simulink model "uav_control_fb_lin_lqr"  (R2023a)
settings: Solver=FixedStepAuto  StartTime=0.0  StopTime=50  FixedStep=1e-3
undefined symbols (not defined in the file): b, d, g, J1, J2, J3, K_lqr, L, m, Matrix_Force2angular_velocity
libraries: simulink x22, hamilton x1, lagrange x1, control_form_NL x1, control_form_NL_forces x1
(part 1 of 2)
settings Model: Creator=Alex  LastModifiedBy=Alex

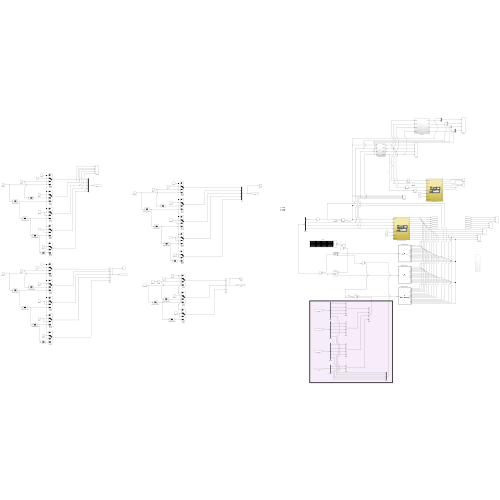
[thumbnail: Simulink's stored preview of the top-level diagram]
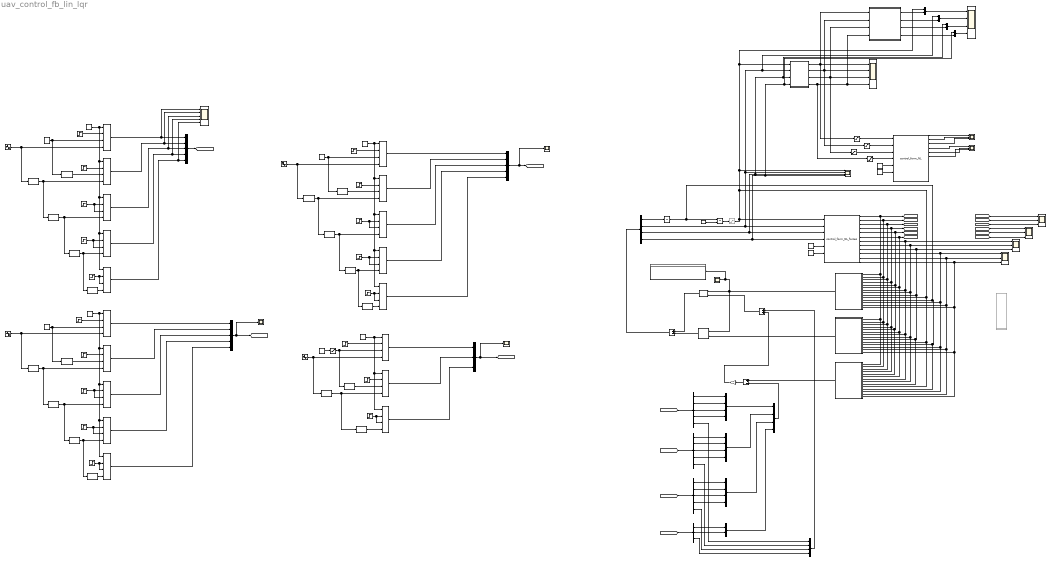
== system uav_control_fb_lin_lqr ==
  note: 1 - step
      | 2 - ramp
      | 3 - else
  Add : Sum  Inputs=+-
  Add1 : Sum  Inputs=+-
  Add2 : Sum
  CNL_AngPos : Scope  NumInputPorts=3
  CNL_AngVel : Scope  NumInputPorts=3
  CNL_LinPos : Scope  NumInputPorts=3
  CNL_LinVel : Scope  NumInputPorts=3
  Constant1 : Constant  Value=[1 0 0 0 1 1 0]
  Constant2 : Constant  Value=[1 1 -1 0 0 0 0 0 0 0 0 0 ]
  Constant3 : Constant  Value=1e-3
  Constant4 : Constant  Value=[1 0 0 0 1 1 0]
  Constant5 : Constant  Value=[1 1 -1 0 0 0 0 0 0 0 0 0 ]
  Demux : Demux
  Demux1 : Demux  Outputs=5
  Demux2 : Demux  Outputs=5
  Demux3 : Demux  Outputs=5
  Demux4 : Demux  Outputs=3
  Discrete Derivative{,1..17} (18 alike) : simulink/Discrete/Discrete Derivative  gainval=1.0  ICPrevScaledInput=0.0  OutMin=[]  OutMax=[]  OutDataType=fixdt(1, 16)  OutScaling=2^-10  DoSatur=off
  Display : Display
  Force2AngularVelocity : Subsystem
  Gain1 : Gain  Gain=-K_lqr  Multiplication=Matrix(K*u)
  Input_psi : Constant
  Input_x : Constant
  Input_y : Constant
  Input_z : Constant
  Integrator : Integrator
  Integrator1 : Integrator  InitialConditionSource=external
  MATLAB Function : MATLAB Function  TreatAsAtomicUnit=on
  MATLAB Function1 : MATLAB Function  TreatAsAtomicUnit=on
  MATLAB Function2 : MATLAB Function  TreatAsAtomicUnit=on
  Matrix Multiply : Product  Multiplication=Matrix(*)
  Multiport Switch{,1..17} (18 alike) : MultiPortSwitch  SaturateOnIntegerOverflow=off  InputSameDT=off
  Mux : Mux  Inputs=5
  Mux1 : Mux  Inputs=5
  Mux{8,10..13} (5 alike) : Mux  Inputs=2
  Mux{2,4,6..7,9} (5 alike) : Mux
  Mux3 : Mux  Inputs=3
  Mux5 : Mux  Inputs=5
  Product : Product  Multiplication=Matrix(*)
  Ramp_psi : simulink/Sources/Ramp  slope=0.2  start=0  InitialOutput=0
  Ramp_x : simulink/Sources/Ramp  slope=1  start=0  InitialOutput=1
  Ramp_y : simulink/Sources/Ramp  slope=1  start=0  InitialOutput=0
  Ramp_z : simulink/Sources/Ramp  slope=-5  start=0  InitialOutput=0
  STEP0_{1..14} (14 alike) : Step  Time=0  After=0  SampleTime=0
  Saturation : Saturate  UpperLimit=pi  LowerLimit=-pi
  Saturation1 : Saturate  Commented=through  UpperLimit=inf  LowerLimit=0
  Saturation{2..5} (4 alike) : Saturate  UpperLimit=1000  LowerLimit=0
  Scope{,2..4} (4 alike) : Scope
  Scope1 : Scope  NumInputPorts=5
  Scope5 : Scope  NumInputPorts=4
  Scope6 : Scope  NumInputPorts=3
  Scope7 : Scope  NumInputPorts=3
  Scope8 : Scope  NumInputPorts=4
  Scope9 : Scope  NumInputPorts=4
  Sine Wave_psi : Sin  SampleTime=0
  Sine Wave_x : Sin  Frequency=0.5  SampleTime=0
  Sine Wave_y : Sin  Amplitude=3  Bias=5  SampleTime=0
  Sine Wave_z : Sin  Amplitude=3  Bias=-5  SampleTime=0
  Step_psi : Step  Time=0  SampleTime=0
  Step_x : Step  Time=0  After=5  SampleTime=0
  Step_y : Step  Time=0  After=5  SampleTime=0
  Step_z : Step  Time=0  After=-7  SampleTime=0
  Subsystem : Subsystem  Commented=on
  Subsystem1 : Subsystem
  control_form_NL : control_form_NL/control_form_NL  SystemSampleTime=-1  VariantActivationTime=update diagram  Latency=0  AutoFrameSizeCalculation=off
  control_form_NL_forces : control_form_NL_forces/control_form_NL_forces  SystemSampleTime=-1  VariantActivationTime=update diagram  Latency=0  AutoFrameSizeCalculation=off
      settings: LibrarySourceBlock=control_form_NL_forces/control_form_NL
  wires:
  control_form_NL_forces/3 -> MATLAB Function2/3(z), MATLAB Function1/3(z), MATLAB Function/3(z), [CNL_z]
  control_form_NL_forces/2 -> MATLAB Function2/2(y), MATLAB Function1/2(y), MATLAB Function/2(y), [CNL_y]
  control_form_NL_forces/1 -> MATLAB Function2/1(x), MATLAB Function1/1(x), MATLAB Function/1(x), [CNL_x]
  control_form_NL_forces/4 -> MATLAB Function2/4(phi), MATLAB Function1/4(phi), MATLAB Function/4(phi), [CNL_phi]
  control_form_NL_forces/5 -> MATLAB Function2/5(theta), MATLAB Function1/5(theta), MATLAB Function/5(theta), [CNL_theta]
  control_form_NL_forces/6 -> MATLAB Function2/6(psi), MATLAB Function1/6(psi), MATLAB Function/6(psi), [CNL_psi]
  [CNL_x] -> CNL_LinPos/1
  [CNL_y] -> CNL_LinPos/2
  [CNL_z] -> CNL_LinPos/3
  [CNL_phi] -> CNL_AngPos/1
  [CNL_theta] -> CNL_AngPos/2
  [CNL_psi] -> CNL_AngPos/3
  control_form_NL_forces/7 -> MATLAB Function2/7(xdot), MATLAB Function1/7(xdot), MATLAB Function/7(xdot), CNL_LinVel/1
  control_form_NL_forces/8 -> MATLAB Function2/8(ydot), MATLAB Function1/8(ydot), MATLAB Function/8(ydot), CNL_LinVel/2
  control_form_NL_forces/9 -> MATLAB Function/9(zdot), MATLAB Function2/9(zdot), MATLAB Function1/9(zdot), CNL_LinVel/3
  control_form_NL_forces/10 -> CNL_AngVel/1, MATLAB Function2/12(p), MATLAB Function1/12(p), MATLAB Function/12(p)
  control_form_NL_forces/11 -> CNL_AngVel/2, MATLAB Function2/13(q), MATLAB Function1/13(q), MATLAB Function/13(q)
  control_form_NL_forces/12 -> CNL_AngVel/3, MATLAB Function2/14(r), MATLAB Function1/14(r), MATLAB Function/14(r)
  Integrator/1 -> MATLAB Function/11(xi), MATLAB Function2/11(xi), MATLAB Function1/11(xi), Integrator1/1  "xi"
  Product/1 -> Add/2  "alpha"
  MATLAB Function1/1(b) -> Product/2
  MATLAB Function/1(delta_inv) -> Display/1, Scope/1, Matrix Multiply/1, Product/1  "beta"
  Matrix Multiply/1 -> Add/1
  Add1/1 -> Gain1/1  "z"
  Gain1/1 -> Add2/2  "v"
  Add/1 -> Demux/1
  Demux/1 -> Integrator/1  "u1_tilde"
  Integrator1/1 -> Saturation1/1  "zeta"
  Step_x/1 -> Multiport Switch/2
  Mux/1 -> [xref]
  Constant1/1 -> control_form_NL_forces/6
  Constant2/1 -> control_form_NL_forces/5
  Constant3/1 -> Integrator1/2
  Mux1/1 -> [yref], Scope2/1
  Step_psi/1 -> Multiport Switch15/2
  Mux3/1 -> [psiref], Scope4/1
  MATLAB Function2/1(transf) -> Add1/1  "z"
  Mux4/1 -> Add1/2
  Ramp_x/1 -> Discrete Derivative/1, Multiport Switch/3
  Sine Wave_x/1 -> Multiport Switch/4, Discrete Derivative1/1
  Input_x/1 -> Multiport Switch4/1, Multiport Switch3/1, Multiport Switch2/1, Multiport Switch1/1, Multiport Switch/1
  STEP0_1/1 -> Multiport Switch1/2
  Discrete Derivative/1 -> Multiport Switch1/3
  Discrete Derivative1/1 -> Multiport Switch1/4, Discrete Derivative2/1
  STEP0_2/1 -> Multiport Switch2/3, Multiport Switch2/2
  Discrete Derivative2/1 -> Multiport Switch2/4, Discrete Derivative3/1
  STEP0_3/1 -> Multiport Switch3/3, Multiport Switch3/2
  Discrete Derivative3/1 -> Multiport Switch3/4, Discrete Derivative4/1
  Discrete Derivative4/1 -> Multiport Switch4/4
  STEP0_4/1 -> Multiport Switch4/3, Multiport Switch4/2
  Multiport Switch/1 -> Mux/1, Scope1/1
  Multiport Switch1/1 -> Mux/2, Scope1/2
  Multiport Switch2/1 -> Mux/3, Scope1/3
  Multiport Switch3/1 -> Mux/4, Scope1/4
  Multiport Switch4/1 -> Scope1/5, Mux/5
  Multiport Switch9/1 -> Mux1/5
  Multiport Switch8/1 -> Mux1/4
  Multiport Switch7/1 -> Mux1/3
  Multiport Switch6/1 -> Mux1/2
  Multiport Switch5/1 -> Mux1/1
  STEP0_8/1 -> Multiport Switch9/2, Multiport Switch9/3
  Discrete Derivative9/1 -> Multiport Switch9/4
  Discrete Derivative8/1 -> Discrete Derivative9/1, Multiport Switch8/4
  STEP0_7/1 -> Multiport Switch8/2, Multiport Switch8/3
  Discrete Derivative7/1 -> Discrete Derivative8/1, Multiport Switch7/4
  STEP0_6/1 -> Multiport Switch7/2, Multiport Switch7/3
  Discrete Derivative6/1 -> Discrete Derivative7/1, Multiport Switch6/4
  Discrete Derivative5/1 -> Multiport Switch6/3
  STEP0_5/1 -> Multiport Switch6/2
  Input_y/1 -> Multiport Switch5/1, Multiport Switch6/1, Multiport Switch7/1, Multiport Switch8/1, Multiport Switch9/1
  Sine Wave_y/1 -> Discrete Derivative6/1, Multiport Switch5/4
  Ramp_y/1 -> Multiport Switch5/3, Discrete Derivative5/1
  Step_y/1 -> Multiport Switch5/2
  Step_z/1 -> Multiport Switch10/2
  Ramp_z/1 -> Discrete Derivative10/1, Multiport Switch10/3
  Sine Wave_z/1 -> Multiport Switch10/4, Discrete Derivative11/1
  Input_z/1 -> Multiport Switch14/1, Multiport Switch13/1, Multiport Switch12/1, Multiport Switch11/1, Multiport Switch10/1
  STEP0_9/1 -> Multiport Switch11/2
  Discrete Derivative10/1 -> Multiport Switch11/3
  Discrete Derivative11/1 -> Multiport Switch11/4, Discrete Derivative12/1
  STEP0_10/1 -> Multiport Switch12/3, Multiport Switch12/2
  Discrete Derivative12/1 -> Multiport Switch12/4, Discrete Derivative13/1
  STEP0_11/1 -> Multiport Switch13/3, Multiport Switch13/2
  Discrete Derivative13/1 -> Multiport Switch13/4, Discrete Derivative14/1
  Discrete Derivative14/1 -> Multiport Switch14/4
  STEP0_12/1 -> Multiport Switch14/3, Multiport Switch14/2
  Multiport Switch10/1 -> Mux5/1
  Multiport Switch11/1 -> Mux5/2
  Multiport Switch12/1 -> Mux5/3
  Multiport Switch13/1 -> Mux5/4
  Multiport Switch14/1 -> Mux5/5
  Mux5/1 -> Scope3/1, [zref]
  Input_psi/1 -> Multiport Switch17/1, Multiport Switch16/1, Multiport Switch15/1
  Ramp_psi/1 -> Saturation/1
  Saturation/1 -> Discrete Derivative15/1, Multiport Switch15/3
  Sine Wave_psi/1 -> Discrete Derivative16/1, Multiport Switch15/4
  STEP0_13/1 -> Multiport Switch16/2
  Discrete Derivative15/1 -> Multiport Switch16/3
  Discrete Derivative16/1 -> Discrete Derivative17/1, Multiport Switch16/4
  STEP0_14/1 -> Multiport Switch17/3, Multiport Switch17/2
  Discrete Derivative17/1 -> Multiport Switch17/4
  [xref] -> Demux1/1
  Demux1/1 -> Mux2/1
  Demux1/2 -> Mux2/2
  Demux1/3 -> Mux2/3
  Demux1/4 -> Mux2/4
  Mux2/1 -> Mux4/1
  Mux6/1 -> Mux4/2
  Demux2/4 -> Mux6/4
  Demux2/3 -> Mux6/3
  Demux2/2 -> Mux6/2
  Demux2/1 -> Mux6/1
  [yref] -> Demux2/1
  [zref] -> Demux3/1
  Demux3/1 -> Mux7/1
  Demux3/2 -> Mux7/2
  Demux3/3 -> Mux7/3
  Demux3/4 -> Mux7/4
  Mux7/1 -> Mux4/3
  [psiref] -> Demux4/1
  Demux4/1 -> Mux8/1
  Demux4/2 -> Mux8/2
  Mux8/1 -> Mux4/4
  Demux4/3 -> Mux9/4
  Demux3/5 -> Mux9/3
  Demux2/5 -> Mux9/2
  Demux1/5 -> Mux9/1
  Mux9/1 -> Add2/1
  Add2/1 -> Matrix Multiply/2
  Constant5/1 -> control_form_NL/5
  Constant4/1 -> control_form_NL/6
  control_form_NL/1 -> Scope6/1
  control_form_NL/2 -> Scope6/2
  control_form_NL/3 -> Scope6/3
  control_form_NL/4 -> Scope7/1
  control_form_NL/5 -> Scope7/2
  control_form_NL/6 -> Scope7/3
  Force2AngularVelocity/1(omega_f) -> Subsystem1/1(omega_f), Scope8/1, Saturation2/1  "front"
  Force2AngularVelocity/2(omega_b) -> Subsystem1/2(omega_b), Scope8/2, Saturation3/1  "back"
  Force2AngularVelocity/3(omega_l) -> Subsystem1/3(omega_l), Scope8/3, Saturation4/1  "left"
  Force2AngularVelocity/4(omega_r) -> Saturation5/1, Subsystem1/4(omega_r), Scope8/4  "right"
  Demux/4 -> control_form_NL_forces/4, Mux13/1, Force2AngularVelocity/4(u4), Scope5/4
  Demux/3 -> control_form_NL_forces/3, Mux12/1, Force2AngularVelocity/3(u3), Scope5/3
  Demux/2 -> control_form_NL_forces/2, Mux11/1, Force2AngularVelocity/2(u2), Scope5/2
  Multiport Switch15/1 -> Mux3/1
  Multiport Switch16/1 -> Mux3/2
  Multiport Switch17/1 -> Mux3/3
  Saturation1/1 -> control_form_NL_forces/1, MATLAB Function2/10(zeta), MATLAB Function1/10(zeta), MATLAB Function/10(zeta), Mux10/1, Force2AngularVelocity/1(u1), Scope5/1
  Subsystem1/1(Thrust) -> Mux10/2
  Subsystem1/2(M1) -> Mux11/2
  Subsystem1/3(M2) -> Mux12/2
  Subsystem1/4(M3) -> Mux13/2
  Mux13/1 -> Scope9/4
  Mux12/1 -> Scope9/3
  Mux11/1 -> Scope9/2
  Mux10/1 -> Scope9/1
  Saturation2/1 -> control_form_NL/1
  Saturation3/1 -> control_form_NL/2
  Saturation4/1 -> control_form_NL/3
  Saturation5/1 -> control_form_NL/4

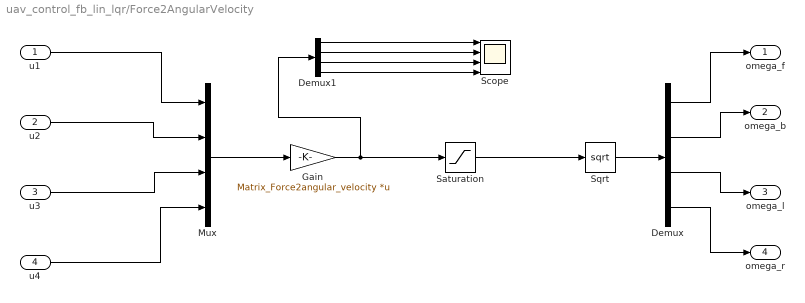
== system uav_control_fb_lin_lqr/Force2AngularVelocity ==
  u1 : Inport
  u2 : Inport  Port=2
  u3 : Inport  Port=3
  u4 : Inport  Port=4
  Demux : Demux
  Demux1 : Demux
  Gain : Gain  Gain=Matrix_Force2angular_velocity  Multiplication=Matrix(K*u)
  Mux : Mux
  Saturation : Saturate  UpperLimit=inf  LowerLimit=0
  Scope : Scope  NumInputPorts=4
  Sqrt : Sqrt
  omega_f : Outport
  omega_b : Outport  Port=2
  omega_l : Outport  Port=3
  omega_r : Outport  Port=4
  wires:
  u3/1 -> Mux/3
  u2/1 -> Mux/2
  u4/1 -> Mux/4
  u1/1 -> Mux/1
  Mux/1 -> Gain/1
  Sqrt/1 -> Demux/1
  Demux/3 -> omega_l/1
  Demux/2 -> omega_b/1
  Demux/4 -> omega_r/1
  Demux/1 -> omega_f/1
  Demux1/1 -> Scope/1
  Demux1/2 -> Scope/2
  Demux1/3 -> Scope/3
  Demux1/4 -> Scope/4
  Gain/1 -> Saturation/1, Demux1/1
  Saturation/1 -> Sqrt/1

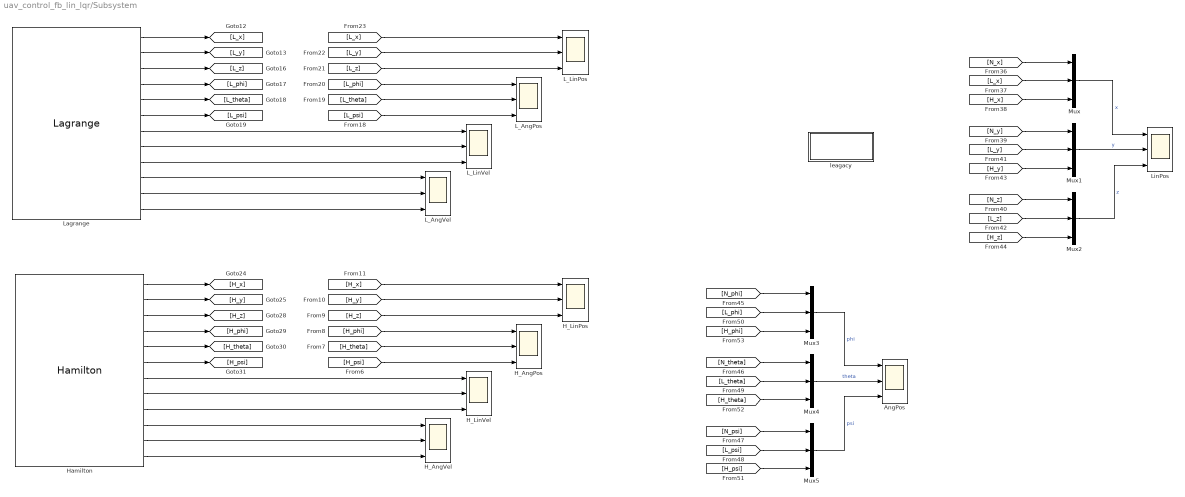
== system uav_control_fb_lin_lqr/Subsystem ==
  AngPos : Scope  NumInputPorts=3
  H_AngPos : Scope  NumInputPorts=3
  H_AngVel : Scope  NumInputPorts=3
  H_LinPos : Scope  NumInputPorts=3
  H_LinVel : Scope  NumInputPorts=3
  Hamilton : hamilton/Hamilton  SystemSampleTime=-1  VariantActivationTime=update diagram  Latency=0  AutoFrameSizeCalculation=off
  L_AngPos : Scope  NumInputPorts=3
  L_AngVel : Scope  NumInputPorts=3
  L_LinPos : Scope  NumInputPorts=3
  L_LinVel : Scope  NumInputPorts=3
  Lagrange : lagrange/Lagrange  SystemSampleTime=-1  VariantActivationTime=update diagram  Latency=0  AutoFrameSizeCalculation=off
  LinPos : Scope  NumInputPorts=3
  Mux{,1..5} (6 alike) : Mux  Inputs=3
  leagacy : Subsystem
  wires:
  Hamilton/2 -> [H_y]
  Mux4/1 -> AngPos/2  "theta"
  [H_theta] -> Mux4/3
  Hamilton/1 -> [H_x]
  Lagrange/11 -> L_AngVel/2
  Mux3/1 -> AngPos/1  "phi"
  [H_theta] -> H_AngPos/2
  Lagrange/4 -> [L_phi]
  Hamilton/6 -> [H_psi]
  Hamilton/10 -> H_AngVel/1
  [H_z] -> H_LinPos/3
  [H_y] -> H_LinPos/2
  Lagrange/10 -> L_AngVel/1
  Lagrange/2 -> [L_y]
  Lagrange/5 -> [L_theta]
  [L_theta] -> Mux4/2
  Hamilton/3 -> [H_z]
  [L_psi] -> Mux5/2
  Lagrange/9 -> L_LinVel/3
  Lagrange/6 -> [L_psi]
  Hamilton/5 -> [H_theta]
  Hamilton/11 -> H_AngVel/2
  Hamilton/9 -> H_LinVel/3
  [L_phi] -> L_AngPos/1
  Lagrange/8 -> L_LinVel/2
  [L_psi] -> L_AngPos/3
  Lagrange/7 -> L_LinVel/1
  [H_psi] -> H_AngPos/3
  [H_psi] -> Mux5/3
  [H_x] -> H_LinPos/1
  [N_psi] -> Mux5/1
  Hamilton/8 -> H_LinVel/2
  [L_x] -> L_LinPos/1
  Hamilton/4 -> [H_phi]
  [L_z] -> L_LinPos/3
  [L_y] -> L_LinPos/2
  Hamilton/12 -> H_AngVel/3
  Mux5/1 -> AngPos/3  "psi"
  Hamilton/7 -> H_LinVel/1
  [H_phi] -> Mux3/3
  Lagrange/12 -> L_AngVel/3
  Lagrange/3 -> [L_z]
  [L_phi] -> Mux3/2
  [N_theta] -> Mux4/1
  [N_phi] -> Mux3/1
  Lagrange/1 -> [L_x]
  [L_theta] -> L_AngPos/2
  [H_phi] -> H_AngPos/1
  [N_x] -> Mux/1
  Mux2/1 -> LinPos/3  "z"
  [H_x] -> Mux/3
  Mux/1 -> LinPos/1  "x"
  [N_z] -> Mux2/1
  [L_x] -> Mux/2
  [L_y] -> Mux1/2
  [L_z] -> Mux2/2
  [N_y] -> Mux1/1
  [H_z] -> Mux2/3
  Mux1/1 -> LinPos/2  "y"
  [H_y] -> Mux1/3

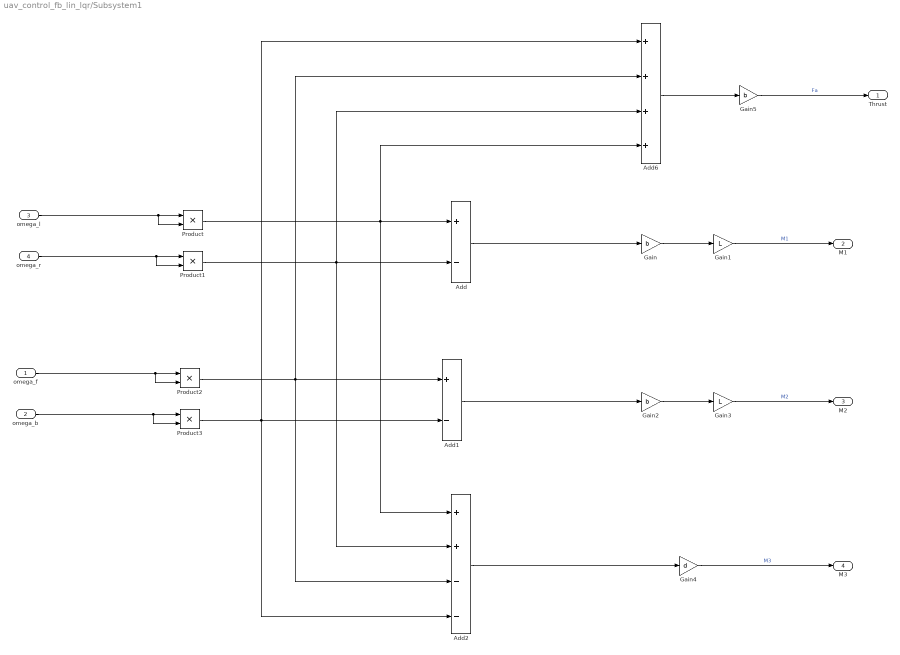
== system uav_control_fb_lin_lqr/Subsystem1 ==
  omega_f : Inport
  omega_b : Inport  Port=2
  omega_l : Inport  Port=3
  omega_r : Inport  Port=4
  Add : Sum  Inputs=+-
  Add1 : Sum  Inputs=+-
  Add2 : Sum  Inputs=++--
  Add6 : Sum  Inputs=++++
  Gain : Gain  Gain=b
  Gain1 : Gain  Gain=L
  Gain2 : Gain  Gain=b
  Gain3 : Gain  Gain=L
  Gain4 : Gain  Gain=d
  Gain5 : Gain  Gain=b
  Product{,1..3} (4 alike) : Product
  Thrust : Outport
  M1 : Outport  Port=2
  M2 : Outport  Port=3
  M3 : Outport  Port=4
  wires:
  Add/1 -> Gain/1
  Gain2/1 -> Gain3/1
  omega_b/1 -> Product3/1, Product3/2
  Product3/1 -> Add6/1, Add2/4, Add1/2
  Product/1 -> Add6/4, Add2/1, Add/1
  omega_f/1 -> Product2/1, Product2/2
  omega_r/1 -> Product1/1, Product1/2
  Add1/1 -> Gain2/1
  Gain4/1 -> M3/1  "M3"
  Add2/1 -> Gain4/1
  Product1/1 -> Add6/3, Add2/2, Add/2
  omega_l/1 -> Product/1, Product/2
  Gain3/1 -> M2/1  "M2"
  Product2/1 -> Add6/2, Add2/3, Add1/1
  Gain/1 -> Gain1/1
  Gain1/1 -> M1/1  "M1"
  Add6/1 -> Gain5/1
  Gain5/1 -> Thrust/1  "Fa"

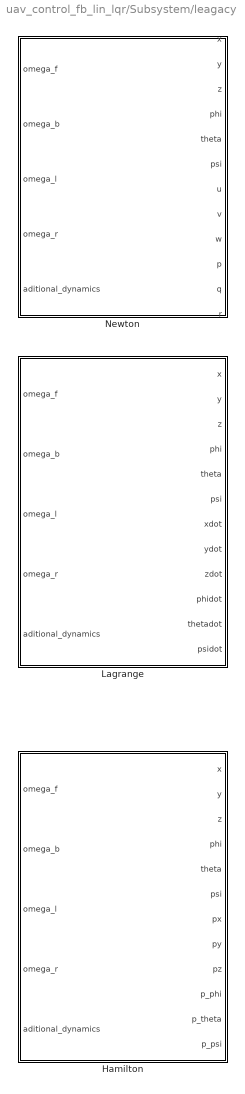
== system uav_control_fb_lin_lqr/Subsystem/leagacy ==
  Hamilton : Subsystem
  Lagrange : Subsystem
  Newton : Subsystem

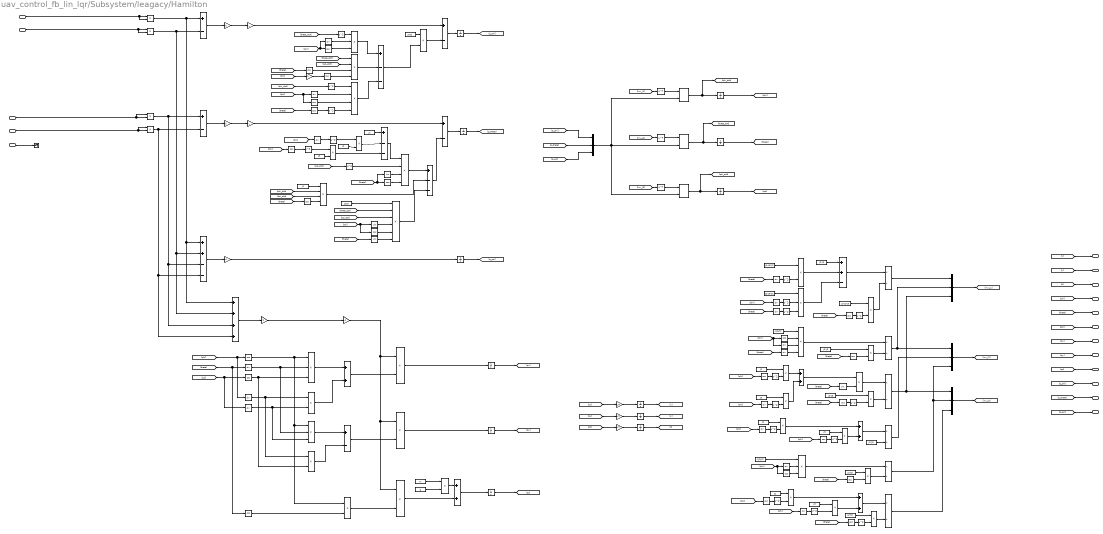
== system uav_control_fb_lin_lqr/Subsystem/leagacy/Hamilton ==
  note: F_thrust
  note: Rotational generalized coordinates (positions)
  note: Translational generalized coordinates (positions)
  note: Translational momentum equations
  note: Rotational momentum equations
  note: Matrix J^(-1) computation
  omega_f : Inport
  omega_b : Inport  Port=2
  omega_l : Inport  Port=3
  omega_r : Inport  Port=4
  aditional_dynamics : Inport  Port=5
  Add{,1,3..4,11} (5 alike) : Sum  Inputs=+-
  Add{10,14,26..28} (5 alike) : Sum
  Add2 : Sum  Inputs=++--
  Add25 : Sum  Inputs=++-
  Add5 : Sum  Inputs=+--
  Add6 : Sum  Inputs=++++
  Add7 : Sum  Inputs=+--
  Add8 : Sum  Inputs=+--
  Constant1 : Constant  Value=J3-J2
  Constant2 : Constant  Value=J1
  Constant{22,26,28,31,34,36} (6 alike) : Constant  Value=J2*J3
  Constant23 : Constant  Value=(J1-J3)*J2
  Constant24 : Constant  Value=(J2-J3)*J1
  Constant25 : Constant  Value=J1*J2*J3
  Constant27 : Constant  Value=-(J2-J3)
  Constant{3,29,32,37} (4 alike) : Constant  Value=J2
  Constant{8,30,33,38} (4 alike) : Constant  Value=J3
  Constant35 : Constant  Value=-(J2-J3)
  Constant4 : Constant  Value=J1
  Constant5 : Constant  Value=J2-J3
  Constant6 : Constant  Value=m
  Constant7 : Constant  Value=g
  Cos{,1,3,5,7,53..55,58,60,63..64,66..67,69} (15 alike) : Trigonometry  Operator=cos
  Cos{4,6,8,50..52,56..57,59,61..62,65,68} (13 alike) : Trigonometry
  Divide{6..11} (6 alike) : Product  Inputs=*/
  Gain : Gain  Gain=b
  Gain1 : Gain  Gain=L
  Gain10 : Gain  Gain=-1
  Gain2 : Gain  Gain=b
  Gain3 : Gain  Gain=L
  Gain4 : Gain  Gain=d
  Gain5 : Gain  Gain=b
  Gain6 : Gain  Gain=1/m
  Gain7 : Gain  Gain=1/m
  Gain8 : Gain  Gain=1/m
  Gain9 : Gain  Gain=2
  Integrator{,1..11} (12 alike) : Integrator
  Matrix Multiply1 : Product  Multiplication=Matrix(*)
  Matrix Multiply2 : Product  Multiplication=Matrix(*)
  Matrix Multiply5 : Product  Multiplication=Matrix(*)
  Mux{,7..9} (4 alike) : Mux  Inputs=3
  Product{,1..4,11..12,14,16..21,44,46..47,49..55,57..59} (27 alike) : Product
  Product10 : Product  Inputs=6
  Product{5,13,15,45,56} (5 alike) : Product  Inputs=3
  Product{6..9,48} (5 alike) : Product  Inputs=4
  Sin{,4,7..10} (6 alike) : Trigonometry
  Sin{1..3,5..6,11..12} (7 alike) : Trigonometry  Operator=cos
  Square{1..6,13..24} (18 alike) : Math  Operator=square
  Terminator : Terminator
  Transpose1 : Math  Operator=transpose
  Transpose2 : Math  Operator=transpose
  Transpose5 : Math  Operator=transpose
  x : Outport
  y : Outport  Port=2
  z : Outport  Port=3
  phi : Outport  Port=4
  theta : Outport  Port=5
  psi : Outport  Port=6
  px : Outport  Port=7
  py : Outport  Port=8
  pz : Outport  Port=9
  p_phi : Outport  Port=10
  p_theta : Outport  Port=11
  p_psi : Outport  Port=12
  wires:
  omega_l/1 -> Product/2, Product/1
  omega_r/1 -> Product1/2, Product1/1
  Product/1 -> Add2/1, Add6/1, Add/1
  Product1/1 -> Add2/2, Add6/2, Add/2
  Add/1 -> Gain/1
  Gain/1 -> Gain1/1
  Gain1/1 -> Add3/1  "M1"
  Gain3/1 -> Add4/1  "M2"
  Gain2/1 -> Gain3/1
  Add1/1 -> Gain2/1
  Product3/1 -> Add6/4, Add2/4, Add1/2
  Product2/1 -> Add6/3, Add2/3, Add1/1
  omega_b/1 -> Product3/1, Product3/2
  omega_f/1 -> Product2/1, Product2/2
  Add2/1 -> Gain4/1
  Gain4/1 -> Integrator/1  "M3"
  Add6/1 -> Gain5/1
  Gain5/1 -> Gain10/1  "Fa"
  [phi] -> Sin9/1, Cos/1
  Cos/1 -> Product17/1, Product15/1, Product13/1
  [theta] -> Sin11/1, Sin8/1
  Sin8/1 -> Product15/2, Product13/2
  [psi] -> Cos1/1, Sin10/1
  Cos1/1 -> Product16/2, Product13/3
  Sin9/1 -> Product16/1, Product14/1
  Sin10/1 -> Product15/3, Product14/2
  Product13/1 -> Add10/1
  Product14/1 -> Add10/2
  Product15/1 -> Add11/1
  Product16/1 -> Add11/2
  Sin11/1 -> Product17/2
  Product17/1 -> Product20/2
  Add11/1 -> Product19/2
  Add10/1 -> Product18/2
  Product20/1 -> Add14/2
  Constant7/1 -> Product12/2
  Product18/1 -> Integrator6/1
  Integrator6/1 -> [px]  "px"
  Product19/1 -> Integrator7/1
  Integrator7/1 -> [py]  "py"
  Add14/1 -> Integrator8/1
  Integrator8/1 -> [pz]  "pz"
  [x] -> x/1
  [y] -> y/1
  [p_psi] -> p_psi/1
  [p_theta] -> p_theta/1
  [p_phi] -> p_phi/1
  [pz] -> pz/1
  [py] -> py/1
  [px] -> px/1
  [psi] -> psi/1
  [theta] -> theta/1
  [phi] -> phi/1
  [z] -> z/1
  aditional_dynamics/1 -> Terminator/1
  Cos55/1 -> Product48/2
  Product46/1 -> Divide6/2
  [phi] -> Cos56/1, Cos55/1
  Square13/1 -> Product44/2
  Add27/1 -> Divide9/1
  Product57/1 -> Divide11/2
  [theta] -> Cos53/1
  Cos53/1 -> Square16/1
  [theta] -> Cos64/1
  Constant23/1 -> Product44/1
  Divide6/1 -> Mux7/1
  Cos58/1 -> Square17/1
  [theta] -> Cos58/1
  Mux7/1 -> [inv_j1]
  Product58/1 -> Add28/1
  Add28/1 -> Divide11/1
  Product59/1 -> Add28/2
  Cos57/1 -> Product48/4
  Add26/1 -> Product50/1
  Cos56/1 -> Product48/3
  Cos67/1 -> Square22/1
  Square22/1 -> Product57/2
  Mux8/1 -> [inv_j2]
  Divide11/1 -> Mux9/3
  Cos69/1 -> Square24/1
  Constant34/1 -> Product55/1
  [theta] -> Cos57/1
  Divide7/1 -> Mux8/1, Mux7/2
  Product52/1 -> Add26/1
  Constant22/1 -> Add25/1
  Constant36/1 -> Product57/1
  [theta] -> Cos50/1
  Constant26/1 -> Product47/1
  Constant35/1 -> Product56/1
  Add25/1 -> Divide6/1
  Cos66/1 -> Product56/3
  Product56/1 -> Divide10/1
  Cos65/1 -> Product56/2
  Cos63/1 -> Square21/1
  [phi] -> Cos61/1
  Constant25/1 -> Product46/1
  Square20/1 -> Product54/2
  Cos62/1 -> Square20/1
  Constant38/1 -> Product59/1
  Divide8/1 -> Mux9/1, Mux7/3
  Product53/1 -> Add27/2
  Product55/1 -> Divide10/2
  Square16/1 -> Product46/2
  Constant24/1 -> Product45/1
  Cos61/1 -> Square19/1
  Product44/1 -> Add25/2
  Square15/1 -> Product45/3
  Constant29/1 -> Product52/1
  Constant33/1 -> Product53/1
  Product51/1 -> Add26/2
  Product49/1 -> Divide8/2
  Product45/1 -> Add25/3
  Square19/1 -> Product51/2
  Constant28/1 -> Product49/1
  Constant32/1 -> Product54/1
  [theta] -> Cos52/1
  [phi] -> Cos68/1
  Cos68/1 -> Square23/1
  Cos51/1 -> Square14/1
  Square14/1 -> Product45/2
  Square18/1 -> Product52/2
  [theta] -> Cos59/1
  Cos54/1 -> Product47/2
  [theta] -> Cos54/1
  Constant31/1 -> Divide9/2
  Constant27/1 -> Product48/1
  Divide10/1 -> Mux9/2, Mux8/3
  [phi] -> Cos63/1
  [phi] -> Cos60/1
  Product54/1 -> Add27/1
  Cos64/1 -> Product55/2
  Constant30/1 -> Product51/1
  Mux9/1 -> [inv_j3]
  Square24/1 -> Product58/2
  Product50/1 -> Divide8/1
  [phi] -> Cos62/1
  Cos59/1 -> Product50/2
  Product47/1 -> Divide7/2
  Cos52/1 -> Square15/1
  [theta] -> Cos67/1
  Square17/1 -> Product49/2
  Product48/1 -> Divide7/1
  Cos50/1 -> Square13/1
  Square23/1 -> Product59/2
  Cos60/1 -> Square18/1
  Square21/1 -> Product53/2
  [phi] -> Cos69/1
  [phi] -> Cos66/1, Cos65/1
  Constant37/1 -> Product58/1
  Divide9/1 -> Mux8/2
  [phi] -> Cos51/1
  Integrator/1 -> [p_psi]
  Integrator1/1 -> [p_theta]
  Integrator2/1 -> [p_phi]
  Integrator4/1 -> [x]
  Integrator3/1 -> [y]
  Integrator5/1 -> [z]
  [px] -> Gain6/1
  Gain6/1 -> Integrator4/1
  [py] -> Gain7/1
  Gain7/1 -> Integrator3/1
  [pz] -> Gain8/1
  Gain8/1 -> Integrator5/1
  Integrator9/1 -> [phi]
  Integrator10/1 -> [theta]
  Integrator11/1 -> [psi]
  [p_phi] -> Mux/1
  [p_theta] -> Mux/2
  [p_psi] -> Mux/3
  Matrix Multiply5/1 -> [phi_dot], Integrator9/1
  Transpose5/1 -> Matrix Multiply5/1
  [inv_j1] -> Transpose5/1
  [inv_j2] -> Transpose1/1
  Transpose1/1 -> Matrix Multiply1/1
  Matrix Multiply1/1 -> [theta_dot], Integrator10/1
  Matrix Multiply2/1 -> [psi_dot], Integrator11/1
  [inv_j3] -> Transpose2/1
  Transpose2/1 -> Matrix Multiply2/1
  Mux/1 -> Matrix Multiply2/2, Matrix Multiply5/2, Matrix Multiply1/2
  Add4/1 -> Integrator1/1
  Add3/1 -> Integrator2/1
  Product4/1 -> Add3/2
  Constant1/1 -> Product4/1
  Add7/1 -> Product4/2
  Product5/1 -> Add7/1
  Product6/1 -> Add7/2
  Product7/1 -> Add7/3
  Add5/1 -> Add4/2
  Product8/1 -> Add5/1
  Product9/1 -> Add5/2
  Product10/1 -> Add5/3
  Add8/1 -> Product8/1
  Constant4/1 -> Product9/1
  Constant5/1 -> Product10/1
  [theta] -> Cos4/1, Cos3/1
  Cos3/1 -> Product8/4
  Cos4/1 -> Product8/3
  [theta_dot] -> Square1/1
  Square1/1 -> Product5/1
  [phi] -> Sin/1, Sin1/1
  Sin1/1 -> Product5/3
  Sin/1 -> Product5/2
  [theta_dot] -> Product6/1
  [psi_dot] -> Product6/2
  [theta] -> Sin2/1
  Sin2/1 -> Product6/3
  Sin3/1 -> Product6/4
  [phi] -> Gain9/1
  Gain9/1 -> Sin3/1
  Square2/1 -> Product7/1
  [phi_dot] -> Square2/1
  [phi] -> Sin4/1, Sin5/1
  Sin4/1 -> Product7/2
  Sin5/1 -> Product7/3
  [theta] -> Sin6/1
  Square3/1 -> Product7/4
  Sin6/1 -> Square3/1
  [psi_dot] -> Square4/1
  Square4/1 -> Product8/2
  [phi_dot] -> Product9/2
  [psi_dot] -> Product9/3
  [theta] -> Cos5/1
  Cos5/1 -> Product9/4
  [theta_dot] -> Product10/2
  [psi_dot] -> Product10/3
  [phi] -> Cos7/1, Cos6/1
  Cos6/1 -> Product10/4
  Cos7/1 -> Product10/5
  Cos8/1 -> Product10/6
  [theta] -> Cos8/1
  Gain10/1 -> Product20/1, Product19/1, Product18/1
  Product12/1 -> Add14/1
  Constant6/1 -> Product12/1
  Constant2/1 -> Add8/1
  Product11/1 -> Add8/2
  Product21/1 -> Add8/3
  Constant3/1 -> Product11/2
  Constant8/1 -> Product21/2
  [phi] -> Sin7/1
  Sin7/1 -> Square5/1
  Square5/1 -> Product11/1
  Sin12/1 -> Square6/1
  [phi] -> Sin12/1
  Square6/1 -> Product21/1

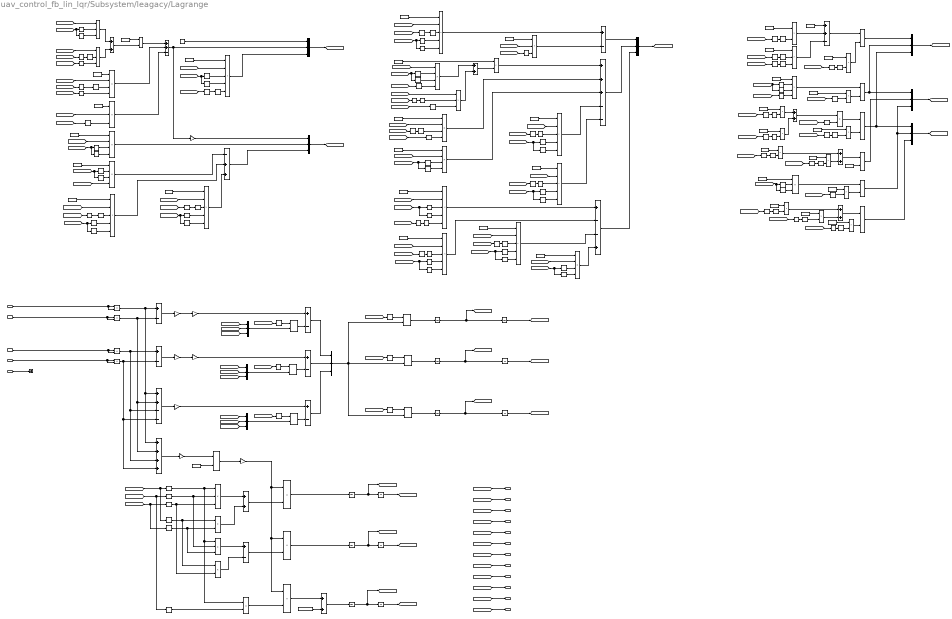
== system uav_control_fb_lin_lqr/Subsystem/leagacy/Lagrange ==
  note: Rotational dynamics
  note: Matrix J^(-1) computation
  note: matrix C computation
  note: Translational dynamics
  omega_f : Inport
  omega_b : Inport  Port=2
  omega_l : Inport  Port=3
  omega_r : Inport  Port=4
  aditional_dynamics : Inport  Port=5
  Add{,1,8,11,14..16} (7 alike) : Sum  Inputs=+-
  Add{3,5,10,12,18..20} (7 alike) : Sum
  Add13 : Sum  Inputs=+--+
  Add17 : Sum  Inputs=++-
  Add2 : Sum  Inputs=++--
  Add4 : Sum  Inputs=++-
  Add6 : Sum  Inputs=++++
  Add7 : Sum  Inputs=-++
  Add9 : Sum  Inputs=+++--
  Constant : Constant  Value=0
  Constant{1,11,14,18} (4 alike) : Constant  Value=J2-J3
  Constant{10,17,20,30,33,38} (6 alike) : Constant  Value=J3
  Constant{4,8,12,15,21} (5 alike) : Constant  Value=J1
  Constant{2,5,7,13} (4 alike) : Constant  Value=J3-J2
  Constant{9,16,19,29,32,37} (6 alike) : Constant  Value=J2
  Constant{22,26,28,31,34,36} (6 alike) : Constant  Value=J2*J3
  Constant23 : Constant  Value=(J1-J3)*J2
  Constant24 : Constant  Value=(J2-J3)*J1
  Constant25 : Constant  Value=J1*J2*J3
  Constant27 : Constant  Value=-(J2-J3)
  Constant3 : Constant  Value=g
  Constant35 : Constant  Value=-(J2-J3)
  Constant6 : Constant  Value=m
  Cos{,1..7,9..10,12,15,17..18,20..21,23..24,28..30,32,34,36,38,40..41,44..45,47,49,53..55,58,60,63..64,66..67,69} (41 alike) : Trigonometry  Operator=cos
  Cos{8,11,13..14,16,19,22,25..27,31,33,35,37,39,42..43,46,48,50..52,56..57,59,61..62,65,68} (29 alike) : Trigonometry
  Divide{,1..6} (7 alike) : Product  Inputs=*/
  Gain : Gain  Gain=b
  Gain1 : Gain  Gain=L
  Gain2 : Gain  Gain=b
  Gain3 : Gain  Gain=L
  Gain4 : Gain  Gain=d
  Gain5 : Gain  Gain=b
  Gain6 : Gain  Gain=-1
  Gain7 : Gain  Gain=-1
  Integrator{,1..11} (12 alike) : Integrator
  Matrix Multiply{1..6} (6 alike) : Product  Multiplication=Matrix(*)
  Mux{,1..9} (10 alike) : Mux  Inputs=3
  Product{,1..4,14,16..20,24,35,37..38,40..46,48..50} (25 alike) : Product
  Product{7,10..11,25,27..28,34,39} (8 alike) : Product  Inputs=4
  Product{9,12,21..22,29..33} (9 alike) : Product  Inputs=5
  Product{5..6,8,13,15,23,26,36,47} (9 alike) : Product  Inputs=3
  Sin{,1,8..10} (5 alike) : Trigonometry
  Sin11 : Trigonometry  Operator=cos
  Square{,1..24} (25 alike) : Math  Operator=square
  Terminator : Terminator
  Transpose{,1..5} (6 alike) : Math  Operator=transpose
  x : Outport
  y : Outport  Port=2
  z : Outport  Port=3
  phi : Outport  Port=4
  theta : Outport  Port=5
  psi : Outport  Port=6
  xdot : Outport  Port=7
  ydot : Outport  Port=8
  zdot : Outport  Port=9
  phidot : Outport  Port=10
  thetadot : Outport  Port=11
  psidot : Outport  Port=12
  wires:
  aditional_dynamics/1 -> Terminator/1
  [z] -> z/1
  [phi] -> phi/1
  [theta] -> theta/1
  [psi] -> psi/1
  [xdot] -> xdot/1
  [ydot] -> ydot/1
  [zdot] -> zdot/1
  [phidot] -> phidot/1
  [thetadot] -> thetadot/1
  [psidot] -> psidot/1
  [y] -> y/1
  [x] -> x/1
  Add10/1 -> Product18/2
  Add11/1 -> Product19/2
  Product17/1 -> Product20/2
  Sin11/1 -> Product17/2
  Product16/1 -> Add11/2
  Product15/1 -> Add11/1
  Product14/1 -> Add10/2
  Product13/1 -> Add10/1
  Sin10/1 -> Product14/2, Product15/3
  Sin9/1 -> Product14/1, Product16/1
  Cos1/1 -> Product13/3, Product16/2
  [psi] -> Sin10/1, Cos1/1
  Sin8/1 -> Product13/2, Product15/2
  [theta] -> Sin8/1, Sin11/1
  Cos/1 -> Product13/1, Product15/1, Product17/1
  [phi] -> Cos/1, Sin9/1
  Divide5/1 -> Gain7/1
  Constant6/1 -> Divide5/2
  Gain5/1 -> Divide5/1  "Fa"
  Add6/1 -> Gain5/1
  Gain4/1 -> Add16/1  "M3"
  Add2/1 -> Gain4/1
  omega_f/1 -> Product2/1, Product2/2
  omega_b/1 -> Product3/1, Product3/2
  Product2/1 -> Add1/1, Add2/3, Add6/3
  Product3/1 -> Add1/2, Add6/4, Add2/4
  Add1/1 -> Gain2/1
  Gain2/1 -> Gain3/1
  Gain3/1 -> Add15/1  "M2"
  Gain1/1 -> Add14/1  "M1"
  Gain/1 -> Gain1/1
  Add/1 -> Gain/1
  Product1/1 -> Add/2, Add6/2, Add2/2
  Product/1 -> Add/1, Add6/1, Add2/1
  omega_r/1 -> Product1/2, Product1/1
  omega_l/1 -> Product/2, Product/1
  Product20/1 -> Add3/1
  Constant3/1 -> Add3/2
  Product18/1 -> Integrator/1
  Product19/1 -> Integrator1/1
  Add3/1 -> Integrator2/1
  Integrator2/1 -> [zdot], Integrator6/1
  Integrator1/1 -> [ydot], Integrator7/1
  Integrator/1 -> [xdot], Integrator8/1
  Integrator8/1 -> [x]
  Integrator7/1 -> [y]
  Integrator6/1 -> [z]
  Integrator3/1 -> [phi]
  Integrator4/1 -> [theta]
  Integrator5/1 -> [psi]
  Integrator9/1 -> Integrator3/1, [phidot]
  Integrator10/1 -> Integrator4/1, [thetadot]
  Integrator11/1 -> Integrator5/1, [psidot]
  Constant/1 -> Mux/1
  Constant1/1 -> Product4/1
  [thetadot] -> Product5/1
  Product4/1 -> Add4/1
  Product5/1 -> Add5/1
  [phi] -> Sin/1, Cos2/1
  Cos2/1 -> Product5/2
  Sin/1 -> Product5/3
  [psidot] -> Product6/1
  [phi] -> Sin1/1
  Sin1/1 -> Square/1
  Square/1 -> Product6/2
  [theta] -> Cos3/1
  Cos3/1 -> Product6/3
  Product6/1 -> Add5/2
  Add5/1 -> Product4/2
  Constant2/1 -> Product7/1
  Add4/1 -> Gain6/1, Mux/2
  [psidot] -> Product7/2
  [phi] -> Cos4/1
  Cos4/1 -> Square1/1
  Square1/1 -> Product7/3
  [theta] -> Cos5/1
  Cos5/1 -> Product7/4
  Product7/1 -> Add4/2
  Constant4/1 -> Product8/1
  [psidot] -> Product8/2
  [theta] -> Cos6/1
  Cos6/1 -> Product8/3
  Product8/1 -> Add4/3
  Product9/1 -> Mux/3
  Constant5/1 -> Product9/1
  [psidot] -> Product9/2
  [phi] -> Cos8/1, Cos7/1
  Cos7/1 -> Product9/3
  Cos8/1 -> Product9/4
  [theta] -> Cos9/1
  Cos9/1 -> Square2/1
  Square2/1 -> Product9/5
  Gain6/1 -> Mux1/1
  Constant7/1 -> Product10/1
  [phidot] -> Product10/2
  [phi] -> Cos11/1, Cos10/1
  Cos10/1 -> Product10/3
  Cos11/1 -> Product10/4
  Product10/1 -> Mux1/2
  Add7/1 -> Mux1/3
  Constant8/1 -> Product11/1
  [theta] -> Cos12/1, Cos13/1
  Cos13/1 -> Product11/2
  Cos12/1 -> Product11/3
  Product11/1 -> Add7/1
  [psidot] -> Product12/2
  Constant9/1 -> Product12/1
  [phi] -> Cos14/1
  Cos14/1 -> Square3/1
  Square3/1 -> Product12/3
  [theta] -> Cos16/1, Cos15/1
  Cos16/1 -> Product12/4
  Cos15/1 -> Product12/5
  Product12/1 -> Add7/2
  Constant10/1 -> Product21/1
  Product21/1 -> Add7/3
  [psidot] -> Product21/2
  Cos17/1 -> Square4/1
  [phi] -> Cos17/1
  Square4/1 -> Product21/3
  Cos18/1 -> Product21/5
  Cos19/1 -> Product21/4
  [theta] -> Cos18/1, Cos19/1
  Add8/1 -> Mux3/1
  Constant11/1 -> Product22/1
  [psidot] -> Product22/2
  [theta] -> Cos20/1
  Cos20/1 -> Square5/1
  Square5/1 -> Product22/3
  [phi] -> Cos22/1, Cos21/1
  Cos22/1 -> Product22/4
  Cos21/1 -> Product22/5
  Product22/1 -> Add8/1
  Product23/1 -> Add8/2
  Constant12/1 -> Product23/1
  [thetadot] -> Product23/2
  Cos23/1 -> Product23/3
  [theta] -> Cos23/1
  Add9/1 -> Mux3/2
  Product24/1 -> Add9/1
  Constant13/1 -> Product24/1
  Add12/1 -> Product24/2
  Product26/1 -> Add12/2
  Product25/1 -> Add12/1
  [thetadot] -> Product25/1
  Cos25/1 -> Product25/2
  [phi] -> Cos24/1, Cos25/1
  Cos24/1 -> Product25/3
  [theta] -> Cos26/1
  Cos26/1 -> Product25/4
  [phidot] -> Product26/1
  [phi] -> Cos27/1
  Cos27/1 -> Square6/1
  Square6/1 -> Product26/2
  [theta] -> Cos28/1
  Cos28/1 -> Product26/3
  Product27/1 -> Add9/2
  Product28/1 -> Add9/3
  Constant14/1 -> Product27/1
  [phidot] -> Product27/2
  Cos29/1 -> Square7/1
  [phi] -> Cos29/1
  Square7/1 -> Product27/3
  [theta] -> Cos30/1
  Cos30/1 -> Product27/4
  Constant15/1 -> Product28/1
  [psidot] -> Product28/2
  Cos31/1 -> Product28/3
  Cos32/1 -> Product28/4
  [theta] -> Cos32/1, Cos31/1
  Product29/1 -> Add9/4
  Product30/1 -> Add9/5
  Constant16/1 -> Product29/1
  Constant17/1 -> Product30/1
  [psidot] -> Product29/2
  [psidot] -> Product30/2
  Square8/1 -> Product29/3
  [phi] -> Cos33/1
  Cos33/1 -> Square8/1
  Square9/1 -> Product30/3
  [phi] -> Cos34/1
  Cos34/1 -> Square9/1
  [theta] -> Cos36/1, Cos35/1
  Cos36/1 -> Product29/5
  Cos35/1 -> Product29/4
  [theta] -> Cos37/1, Cos38/1
  Cos37/1 -> Product30/4
  Cos38/1 -> Product30/5
  Add13/1 -> Mux3/3
  Product31/1 -> Add13/1
  Product32/1 -> Add13/2
  Product33/1 -> Add13/3
  Product34/1 -> Add13/4
  Constant18/1 -> Product31/1
  [phidot] -> Product31/2
  Cos40/1 -> Product31/4
  Cos39/1 -> Product31/3
  [phi] -> Cos39/1, Cos40/1
  Cos41/1 -> Square10/1
  [theta] -> Cos41/1
  Square10/1 -> Product31/5
  Constant19/1 -> Product32/1
  [thetadot] -> Product32/2
  Cos42/1 -> Square11/1
  Square11/1 -> Product32/3
  [phi] -> Cos42/1
  [theta] -> Cos44/1, Cos43/1
  Cos44/1 -> Product32/5
  Cos43/1 -> Product32/4
  Constant20/1 -> Product33/1
  [thetadot] -> Product33/2
  Cos45/1 -> Square12/1
  [phi] -> Cos45/1
  Square12/1 -> Product33/3
  [theta] -> Cos47/1, Cos46/1
  Cos47/1 -> Product33/5
  Cos46/1 -> Product33/4
  Constant21/1 -> Product34/1
  [thetadot] -> Product34/2
  [theta] -> Cos49/1, Cos48/1
  Cos49/1 -> Product34/4
  Cos48/1 -> Product34/3
  Mux5/1 -> Matrix Multiply2/2
  [phidot] -> Mux5/1
  [thetadot] -> Mux5/2
  [psidot] -> Mux5/3
  Matrix Multiply3/1 -> Integrator10/1
  Matrix Multiply4/1 -> Integrator9/1
  Matrix Multiply5/1 -> Integrator11/1
  Mux/1 -> [c1]
  Mux1/1 -> [c2]
  Mux3/1 -> [c3]
  [c1] -> Transpose/1
  Matrix Multiply2/1 -> Add14/2
  Matrix Multiply6/1 -> Add15/2
  [c2] -> Transpose1/1
  [psidot] -> Mux2/3
  [thetadot] -> Mux2/2
  [phidot] -> Mux2/1
  Mux2/1 -> Matrix Multiply6/2
  Mux4/1 -> Matrix Multiply1/2
  [phidot] -> Mux4/1
  [thetadot] -> Mux4/2
  [psidot] -> Mux4/3
  [c3] -> Transpose2/1
  Matrix Multiply1/1 -> Add16/2
  Add15/1 -> Mux6/2
  Add14/1 -> Mux6/1
  Add16/1 -> Mux6/3
  Mux6/1 -> Matrix Multiply5/2, Matrix Multiply3/2, Matrix Multiply4/2
  Transpose/1 -> Matrix Multiply2/1
  Transpose1/1 -> Matrix Multiply6/1
  Transpose2/1 -> Matrix Multiply1/1
  Add17/1 -> Divide/1
  Constant22/1 -> Add17/1
  Product35/1 -> Add17/2
  Constant23/1 -> Product35/1
  [theta] -> Cos50/1
  Cos50/1 -> Square13/1
  Square13/1 -> Product35/2
  Constant24/1 -> Product36/1
  Product36/1 -> Add17/3
  Cos51/1 -> Square14/1
  [phi] -> Cos51/1
  Square14/1 -> Product36/2
  [theta] -> Cos52/1
  Cos52/1 -> Square15/1
  Square15/1 -> Product36/3
  Product37/1 -> Divide/2
  Constant25/1 -> Product37/1
  Cos53/1 -> Square16/1
  [theta] -> Cos53/1
  Square16/1 -> Product37/2
  Divide/1 -> Mux7/1
  Constant26/1 -> Product38/1
  Product38/1 -> Divide1/2
  Divide1/1 -> Mux8/1, Mux7/2
  [theta] -> Cos54/1
  Cos54/1 -> Product38/2
  Constant27/1 -> Product39/1
  [phi] -> Cos56/1, Cos55/1
  Cos55/1 -> Product39/2
  Cos56/1 -> Product39/3
  Cos57/1 -> Product39/4
  [theta] -> Cos57/1
  Product39/1 -> Divide1/1
  Product40/1 -> Divide2/2
  Divide2/1 -> Mux9/1, Mux7/3
  Constant28/1 -> Product40/1
  [theta] -> Cos58/1
  Cos58/1 -> Square17/1
  Square17/1 -> Product40/2
  Product41/1 -> Divide2/1
  [theta] -> Cos59/1
  Cos59/1 -> Product41/2
  Add18/1 -> Product41/1
  Product42/1 -> Add18/2
  Product43/1 -> Add18/1
  Constant29/1 -> Product43/1
  Constant30/1 -> Product42/1
  Cos60/1 -> Square18/1
  Square18/1 -> Product43/2
  [phi] -> Cos60/1
  Constant31/1 -> Divide3/2
  Add19/1 -> Divide3/1
  [phi] -> Cos61/1
  Cos61/1 -> Square19/1
  Square19/1 -> Product42/2
  Product45/1 -> Add19/1
  Product44/1 -> Add19/2
  Constant32/1 -> Product45/1
  Constant33/1 -> Product44/1
  Cos62/1 -> Square20/1
  [phi] -> Cos62/1
  Square20/1 -> Product45/2
  Square21/1 -> Product44/2
  [phi] -> Cos63/1
  Cos63/1 -> Square21/1
  Divide3/1 -> Mux8/2
  Product46/1 -> Divide4/2
  Divide4/1 -> Mux9/2, Mux8/3
  Constant34/1 -> Product46/1
  [theta] -> Cos64/1
  Cos64/1 -> Product46/2
  Product47/1 -> Divide4/1
  Constant35/1 -> Product47/1
  [phi] -> Cos66/1, Cos65/1
  Cos65/1 -> Product47/2
  Cos66/1 -> Product47/3
  Product48/1 -> Divide6/2
  Constant36/1 -> Product48/1
  Cos67/1 -> Square22/1
  [theta] -> Cos67/1
  Square22/1 -> Product48/2
  Divide6/1 -> Mux9/3
  Add20/1 -> Divide6/1
  Product50/1 -> Add20/2
  Product49/1 -> Add20/1
  Constant37/1 -> Product49/1
  [phi] -> Cos68/1
  Cos68/1 -> Square23/1
  Cos69/1 -> Square24/1
  [phi] -> Cos69/1
  Square24/1 -> Product49/2
  Square23/1 -> Product50/2
  Constant38/1 -> Product50/1
  Mux7/1 -> [inv_j1]
  Mux8/1 -> [inv_j2]
  Mux9/1 -> [inv_j3]
  Transpose3/1 -> Matrix Multiply4/1
  [inv_j1] -> Transpose3/1
  [inv_j2] -> Transpose4/1
  Transpose4/1 -> Matrix Multiply3/1
  [inv_j3] -> Transpose5/1
  Transpose5/1 -> Matrix Multiply5/1
  Gain7/1 -> Product18/1, Product19/1, Product20/1
  [psidot] -> Product11/4

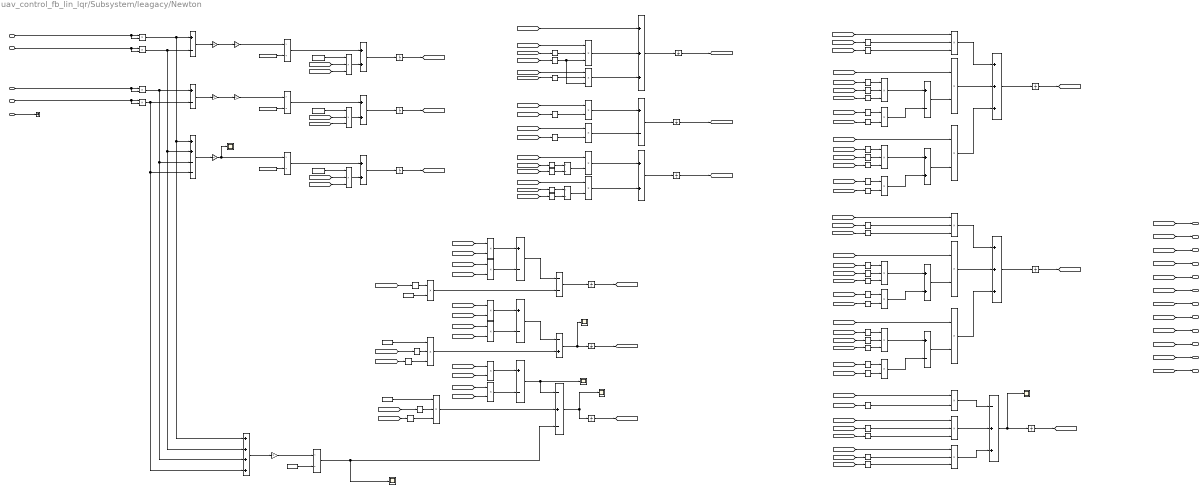
== system uav_control_fb_lin_lqr/Subsystem/leagacy/Newton ==
  note: Inertial velocities in terms of body fixed velocities
      | Translational velocities
  note: Newton's second law
      | Translational accelerations
  note: Euler Angles
      | Rotational velocities
  note: Euler equations of motion
      | Rotational accelerations
  omega_f : Inport
  omega_b : Inport  Port=2
  omega_l : Inport  Port=3
  omega_r : Inport  Port=4
  aditional_dynamics : Inport  Port=5
  Add{,1,8,15..17,19,23} (8 alike) : Sum  Inputs=+-
  Add12 : Sum  Inputs=--
  Add13 : Sum  Inputs=-+
  Add14 : Sum  Inputs=-+-
  Add18 : Sum  Inputs=+++
  Add2 : Sum  Inputs=++--
  Add{3..5,9,20,22} (6 alike) : Sum
  Add21 : Sum  Inputs=+++
  Add24 : Sum  Inputs=-++
  Add6 : Sum  Inputs=++++
  Add7 : Sum  Inputs=+++
  Constant : Constant  Value=J1
  Constant1 : Constant  Value=J2
  Constant2 : Constant  Value=J3
  Constant3 : Constant  Value=(J2-J3)/J1
  Constant4 : Constant  Value=(J3-J1)/J2
  Constant5 : Constant  Value=(J1-J2)/J3
  Constant6 : Constant  Value=m
  Constant7 : Constant  Value=g
  Constant8 : Constant  Value=g
  Constant9 : Constant  Value=g
  Cos10 : Trigonometry
  Cos{2..8,11..12} (9 alike) : Trigonometry  Operator=cos
  Cos13 : Trigonometry
  Cos9 : Trigonometry
  Divide{,1..5} (6 alike) : Product  Inputs=*/
  Gain : Gain  Gain=b
  Gain1 : Gain  Gain=L
  Gain2 : Gain  Gain=b
  Gain3 : Gain  Gain=L
  Gain4 : Gain  Gain=d
  Gain5 : Gain  Gain=b
  Integrator{,1..11} (12 alike) : Integrator
  Product{,1..3,9..13,21..26,28..29,31,33,35..36,38,40,42} (24 alike) : Product
  Product{4..8,14..15,27,30,32,34,37,39,41,43} (15 alike) : Product  Inputs=3
  Scope{,1,3..6} (6 alike) : Scope
  Sin{,3..4,8,10,12..19,21..22,24..25} (17 alike) : Trigonometry
  Sin{1..2,5..7,9,11,20,23,26..29} (13 alike) : Trigonometry  Operator=cos
  Tan : Trigonometry  Operator=tan
  Terminator : Terminator
  x : Outport
  y : Outport  Port=2
  z : Outport  Port=3
  phi : Outport  Port=4
  theta : Outport  Port=5
  psi : Outport  Port=6
  u : Outport  Port=7
  v : Outport  Port=8
  w : Outport  Port=9
  p : Outport  Port=10
  q : Outport  Port=11
  r : Outport  Port=12
  wires:
  omega_l/1 -> Product/1, Product/2
  omega_r/1 -> Product1/1, Product1/2
  Product/1 -> Add2/1, Add6/1, Add/1
  Product1/1 -> Add2/2, Add6/2, Add/2
  Add/1 -> Gain/1
  Gain/1 -> Gain1/1
  Gain1/1 -> Divide/1  "M1"
  Gain3/1 -> Divide1/1  "M2"
  Gain2/1 -> Gain3/1
  Add1/1 -> Gain2/1
  Product3/1 -> Add2/4, Add6/4, Add1/2
  Product2/1 -> Add6/3, Add2/3, Add1/1
  omega_b/1 -> Product3/2, Product3/1
  omega_f/1 -> Product2/2, Product2/1
  Add2/1 -> Gain4/1
  Gain4/1 -> Scope3/1, Divide2/1  "M3"
  Constant/1 -> Divide/2
  Constant1/1 -> Divide1/2
  Constant2/1 -> Divide2/2
  Divide/1 -> Add3/1
  Divide1/1 -> Add4/1
  Divide2/1 -> Add5/1
  Integrator/1 -> [p]  "p"
  Integrator1/1 -> [q]  "q"
  Integrator2/1 -> [r]  "r"
  Product4/1 -> Add3/2
  Product5/1 -> Add4/2
  Product6/1 -> Add5/2
  Constant3/1 -> Product4/1
  Constant4/1 -> Product5/1
  Constant5/1 -> Product6/1
  Add3/1 -> Integrator/1
  Add4/1 -> Integrator1/1
  Add5/1 -> Integrator2/1
  [q] -> Product4/2
  [r] -> Product4/3
  [r] -> Product5/2
  [p] -> Product5/3
  [p] -> Product6/2
  [q] -> Product6/3
  Add6/1 -> Gain5/1
  Gain5/1 -> Divide5/1  "Fa"
  Integrator3/1 -> [phi]
  Integrator4/1 -> [theta]
  Integrator5/1 -> [psi]
  Add7/1 -> Integrator3/1
  Add8/1 -> Integrator4/1
  Add9/1 -> Integrator5/1
  [p] -> Add7/1
  Product7/1 -> Add7/2
  Product8/1 -> Add7/3
  [phi] -> Sin/1
  Sin/1 -> Product7/2
  [theta] -> Tan/1
  Tan/1 -> Product8/3, Product7/3
  [phi] -> Sin1/1
  Sin1/1 -> Product8/2
  [r] -> Product8/1
  [phi] -> Sin2/1
  Sin2/1 -> Product9/2
  [q] -> Product9/1
  Product9/1 -> Add8/1
  Product10/1 -> Add8/2
  [r] -> Product10/1
  [phi] -> Sin3/1
  Sin3/1 -> Product10/2
  Divide3/1 -> Product11/2
  [q] -> Product11/1
  [r] -> Product12/1
  [phi] -> Sin4/1
  Sin4/1 -> Divide3/1
  Sin5/1 -> Divide3/2
  [theta] -> Sin5/1
  Product11/1 -> Add9/1
  Product12/1 -> Add9/2
  Divide4/1 -> Product12/2
  [phi] -> Sin6/1
  Sin6/1 -> Divide4/1
  Sin7/1 -> Divide4/2
  [theta] -> Sin7/1
  Constant6/1 -> Divide5/2
  Product14/1 -> Add13/2
  Product13/1 -> Add12/2
  Product21/1 -> Add15/1
  Product22/1 -> Add15/2
  Add15/1 -> Add12/1
  Add12/1 -> Integrator6/1
  Integrator6/1 -> [u]  "u"
  Add13/1 -> Scope4/1, Integrator7/1
  Integrator7/1 -> [v]  "v"
  Add14/1 -> Integrator8/1, Scope5/1
  Integrator8/1 -> [w]  "w"
  [w] -> Product21/2
  [q] -> Product21/1
  [r] -> Product22/1
  [v] -> Product22/2
  Add16/1 -> Add13/1
  [w] -> Product24/2
  [p] -> Product24/1
  [r] -> Product23/1
  [u] -> Product23/2
  Product24/1 -> Add16/2
  Product23/1 -> Add16/1
  Product25/1 -> Add17/1
  Product26/1 -> Add17/2
  [v] -> Product25/2
  [p] -> Product25/1
  [q] -> Product26/1
  [u] -> Product26/2
  Add17/1 -> Add14/1, Scope/1
  Product28/1 -> Add18/2
  Product27/1 -> Add18/1
  Product29/1 -> Add18/3
  [u] -> Product27/1
  [v] -> Product28/1
  [w] -> Product29/1
  Add18/1 -> Integrator9/1
  Integrator9/1 -> [x]
  Add19/1 -> Product28/2
  Add20/1 -> Product29/2
  [theta] -> Cos2/1
  Cos2/1 -> Product27/2
  [psi] -> Cos3/1
  Cos3/1 -> Product27/3
  Product30/1 -> Add19/1
  Sin12/1 -> Product30/1
  [phi] -> Sin12/1
  Sin13/1 -> Product30/2
  [theta] -> Sin13/1
  [psi] -> Cos4/1
  Cos4/1 -> Product30/3
  Product31/1 -> Add19/2
  Sin14/1 -> Product31/2
  [phi] -> Cos5/1
  [psi] -> Sin14/1
  Cos5/1 -> Product31/1
  Product32/1 -> Add20/1
  Product33/1 -> Add20/2
  Cos6/1 -> Product32/1
  Sin15/1 -> Product32/2
  Cos7/1 -> Product32/3
  [phi] -> Cos6/1
  [theta] -> Sin15/1
  [psi] -> Cos7/1
  Sin16/1 -> Product33/1
  Sin17/1 -> Product33/2
  [phi] -> Sin16/1
  [psi] -> Sin17/1
  [psi] -> Sin23/1
  [phi] -> Sin22/1
  Sin23/1 -> Product40/2
  Sin22/1 -> Product40/1
  [psi] -> Cos13/1
  [theta] -> Sin21/1
  [phi] -> Cos12/1
  Cos13/1 -> Product39/3
  Sin21/1 -> Product39/2
  Cos12/1 -> Product39/1
  Product40/1 -> Add23/2
  Product39/1 -> Add23/1
  Cos11/1 -> Product38/1
  [psi] -> Sin20/1
  [phi] -> Cos11/1
  Sin20/1 -> Product38/2
  Product38/1 -> Add22/2
  Cos10/1 -> Product37/3
  [psi] -> Cos10/1
  [theta] -> Sin19/1
  Sin19/1 -> Product37/2
  [phi] -> Sin18/1
  Sin18/1 -> Product37/1
  Product37/1 -> Add22/1
  Cos9/1 -> Product34/3
  [psi] -> Cos9/1
  Cos8/1 -> Product34/2
  [theta] -> Cos8/1
  Add23/1 -> Product36/2
  Add22/1 -> Product35/2
  Integrator10/1 -> [y]
  Add21/1 -> Integrator10/1
  [w] -> Product36/1
  [v] -> Product35/1
  [u] -> Product34/1
  Product36/1 -> Add21/3
  Product34/1 -> Add21/1
  Product35/1 -> Add21/2
  Add24/1 -> Scope6/1, Integrator11/1
  Integrator11/1 -> [z]
  Product41/1 -> Add24/3
  Product43/1 -> Add24/2
  Product42/1 -> Add24/1
  [theta] -> Sin24/1
  [u] -> Product42/1
  Sin24/1 -> Product42/2
  [v] -> Product43/1
  [w] -> Product41/1
  [phi] -> Sin27/1
  [theta] -> Sin28/1
  [phi] -> Sin25/1
  [theta] -> Sin26/1
  Sin25/1 -> Product43/2
  Sin26/1 -> Product43/3
  Sin27/1 -> Product41/2
  Sin28/1 -> Product41/3
  [x] -> x/1
  [y] -> y/1
  [r] -> r/1
  [q] -> q/1
  [p] -> p/1
  [w] -> w/1
  [v] -> v/1
  [u] -> u/1
  [psi] -> psi/1
  [theta] -> theta/1
  [phi] -> phi/1
  [z] -> z/1
  aditional_dynamics/1 -> Terminator/1
  Divide5/1 -> Scope1/1, Add14/3
  [q] -> Product7/1
  Constant7/1 -> Product13/2
  [theta] -> Sin8/1
  Sin8/1 -> Product13/1
  Constant8/1 -> Product14/1
  [theta] -> Sin9/1
  Sin9/1 -> Product14/2
  [phi] -> Sin10/1
  Sin10/1 -> Product14/3
  Product15/1 -> Add14/2
  Constant9/1 -> Product15/1
  [theta] -> Sin11/1
  Sin11/1 -> Product15/2
  Sin29/1 -> Product15/3
  [phi] -> Sin29/1

== matlab function uav_control_fb_lin_lqr/MATLAB Function1 ==
  data: x input; b output; y input; z input; phi input; theta input; psi input; xdot input; ydot input; zdot input; zeta input; xi input; p input; q input; r input
function b = b_function(x,y,z,phi,theta,psi,xdot,ydot,zdot,zeta,xi,p,q,r)

% prep
m=1.88;
g=9.81;
J1=1.453e-2;
J2=1.453e-2;
J3=2.884e-2;

input1=0;
input2=0;
input3=0;
input4=0;

sphi=sin(phi);
cphi=cos(phi);
stheta=sin(theta);
ctheta=cos(theta);
spsi=sin(psi);
cpsi=cos(psi);

% model dynamics
phi_dot=p+q*(sin(phi)*tan(theta))+r*(cos(phi)*tan(theta));
theta_dot=q*cos(phi)-r*sin(phi);
psi_dot=q*sin(phi)/cos(theta)+r*cos(phi)/cos(theta);


zeta_dot=xi;
xi_dot=input1;

p_dot=(J2-J3)/J1*q*r+1/J1*input2;
q_dot=(J3-J1)/J2*r*p+1/J2*input3;
r_dot=(J1-J2)/J3*p*q+1/J3*input4;

%others
phi_d_dot=p_dot+q_dot*sphi*tan(theta)+phi_dot*q*cphi*tan(theta)+theta_dot*q*sphi/(ctheta^2)+...
r_dot*cphi*tan(theta)-phi_dot*r*sphi*tan(theta)+theta_dot*r*cphi/(ctheta^2);

theta_d_dot=q_dot*cphi-phi_dot*q*sphi-r_dot*sphi-r*phi_dot*cphi;

psi_d_dot=q_dot*sphi/ctheta+q/(ctheta^2)*(phi_dot*cphi*ctheta+theta_dot*sphi*stheta)+...
r_dot*cphi/ctheta+r/(ctheta^2)*(-phi_dot*sphi*ctheta+theta_dot*cphi*stheta);

%%%--------------------------------------------------------------------------------------

%x

Cx=cphi*stheta*cpsi+sphi*spsi;

Cx_dot=-phi_dot*sphi*stheta*cpsi+theta_dot*cphi*ctheta*cpsi-psi_dot*cphi*stheta*spsi...
+phi_dot*cphi*spsi+psi_dot*sphi*cpsi;

Cx_d_dot=psi_d_dot*(-sphi*stheta*cpsi+cphi*spsi)+theta_d_dot*cphi*ctheta*cpsi...
+psi_d_dot*(-cphi*stheta*spsi+sphi*cpsi)-cphi*stheta*cpsi*(phi_dot^2+theta_dot^2+psi_dot^2)...
-2*phi_dot*theta_dot*sphi*ctheta*cpsi+2*phi_dot*psi_dot*sphi*stheta*spsi...
-2*theta_dot*psi_dot*cphi*ctheta*spsi-sphi*spsi*(phi_dot^2+psi_dot^2)+2*phi_dot*psi_dot*cphi*cpsi;

x_4dots=-1/m*(input1*Cx+2*xi*Cx_dot+zeta*Cx_d_dot); % Lf4h1(x)
LgLf3h1=-1/m*[Cx,...
    1/J1*zeta*(-sphi*stheta*cpsi+cphi*spsi),...
    1/J2*zeta*((-sphi*stheta*cpsi+cphi*spsi)*sphi*tan(theta)+cphi*ctheta*cpsi*cphi+...
    (-cphi*stheta*spsi+sphi*cpsi)*sphi/ctheta),...
    1/J3*zeta*((-sphi*stheta*cpsi+cphi*spsi)*cphi*tan(theta)-cphi*ctheta*cpsi*sphi+...
    (-cphi*stheta*spsi+sphi*cpsi)*cphi/ctheta)];

%y

Cy=cphi*stheta*spsi-sphi*cpsi;

Cy_dot=-phi_dot*sphi*stheta*spsi+theta_dot*cphi*ctheta*spsi+psi_dot*cphi*stheta*cpsi...
-phi_dot*cphi*cpsi+psi_dot*sphi*spsi;

Cy_d_dot=phi_d_dot*(-sphi*stheta*spsi-cphi*cpsi)+theta_d_dot*cphi*ctheta*spsi...
+psi_d_dot*(cphi*stheta*cpsi+sphi*spsi)-cphi*stheta*spsi*(phi_dot^2+theta_dot^2+psi_dot^2)...
-2*phi_dot*theta_dot*sphi*ctheta*spsi-2*phi_dot*psi_dot*sphi*stheta*cpsi...
+2*theta_dot*psi_dot*cphi*ctheta*cpsi+sphi*cpsi*(phi_dot^2+psi_dot^2)+2*phi_dot*psi_dot*cphi*spsi;

y_4dots=-1/m*(input1*Cy+2*xi*Cy_dot+zeta*Cy_d_dot);
LgLf3h2=-1/m*[Cy,...
    1/J1*zeta*(-sphi*stheta*spsi-cphi*cpsi),...
    1/J2*zeta*((-sphi*stheta*spsi-cphi*cpsi)*sphi*tan(theta)+cphi*ctheta*spsi*cphi+...
    (cphi*stheta*cpsi+sphi*spsi)*sphi/ctheta),...
    1/J3*zeta*((-sphi*stheta*spsi-cphi*cpsi)*cphi*tan(theta)-cphi*ctheta*spsi*sphi+...
    (cphi*stheta*cpsi+sphi*spsi)*cphi/ctheta)];
%z
Cz=cphi*ctheta;

Cz_dot=-phi_dot*sphi*ctheta-theta_dot*cphi*stheta;

Cz_d_dot=-phi_d_dot*sphi*ctheta-phi_dot^2*cphi*ctheta+2*phi_dot*theta_dot*sphi*stheta...
    -theta_d_dot*cphi*stheta-theta_dot^2*cphi*ctheta;

z_4dots=-1/m*(input1*Cz+2*xi*Cz_dot+zeta*Cz_d_dot);
LgLf3h3=-1/m*[Cz,...
    1/J1*zeta*(-sphi*ctheta),...
    1/J2*zeta*(-sphi*ctheta*sphi*tan(theta)-cphi*stheta*cphi),...
    1/J3*zeta*(-sphi*ctheta*cphi*tan(theta)+cphi*stheta*sphi)];

%psi

%psi_d_dot is defined above
LgLf1h4=[0,...
    0,...
    1/J2*sphi/ctheta,...
    1/J3*cphi/ctheta];
b=[x_4dots;y_4dots;z_4dots;psi_d_dot];
